simulink model "suduZB"  (R2021a)
settings: Solver=FixedStepAuto  StartTime=0.0  StopTime=20.0  FixedStep=0.01  RelTol=1e-3
libraries: simulink x10
settings Model: Creator=Wang Xu  LastModifiedBy=Wang Xu

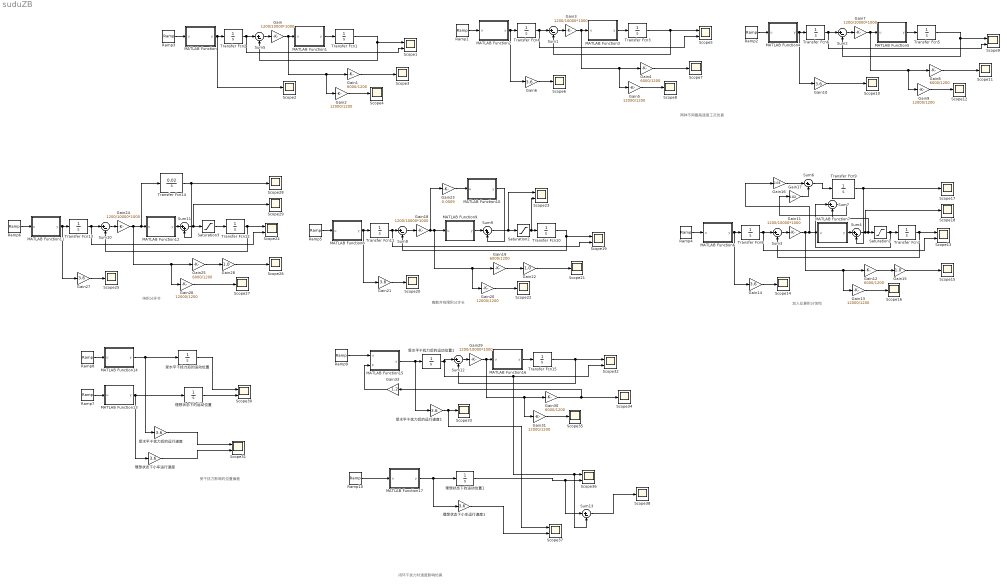
== system suduZB ==
  note: 加入反算积分饱和
  note: 离散并有限积分步长
  note: 纯积分环节
  note: 两种不同最高速度工况仿真
  note: 受干扰力影响的位置偏差
  note: 闭环干扰力对速度影响仿真
  Gain{,3,7,11,18,24,29} (7 alike) : Gain  Gain=1200/10000*1000
  Gain{1,4,8,12,19,25,30} (7 alike) : Gain  Gain=6000/1200
  Gain{6,10,14,21,27} (5 alike) : Gain  Gain=3.6
  Gain{2,5,9,13,20,26,31} (7 alike) : Gain  Gain=12000/1200
  Gain15 : Gain  Gain=1.0
  Gain16 : Gain  Gain=0.03
  Gain17 : Gain  Gain=0.02
  Gain22 : Gain  Gain=1.0
  Gain23 : Gain  Gain=0.0009
  Gain28 : Gain  Gain=1.0
  Gain33 : Gain  Gain=1.2
  MATLAB Function : MATLAB Function  TreatAsAtomicUnit=on
  MATLAB Function1 : MATLAB Function  TreatAsAtomicUnit=on
  MATLAB Function10 : MATLAB Function  TreatAsAtomicUnit=on
  MATLAB Function11 : MATLAB Function  TreatAsAtomicUnit=on
  MATLAB Function12 : MATLAB Function  TreatAsAtomicUnit=on
  MATLAB Function13 : MATLAB Function  TreatAsAtomicUnit=on
  MATLAB Function14 : MATLAB Function  TreatAsAtomicUnit=on
  MATLAB Function15 : MATLAB Function  TreatAsAtomicUnit=on
  MATLAB Function16 : MATLAB Function  TreatAsAtomicUnit=on
  MATLAB Function17 : MATLAB Function  TreatAsAtomicUnit=on
  MATLAB Function2 : MATLAB Function  TreatAsAtomicUnit=on
  MATLAB Function3 : MATLAB Function  TreatAsAtomicUnit=on
  MATLAB Function4 : MATLAB Function  TreatAsAtomicUnit=on
  MATLAB Function5 : MATLAB Function  TreatAsAtomicUnit=on
  MATLAB Function6 : MATLAB Function  TreatAsAtomicUnit=on
  MATLAB Function7 : MATLAB Function  TreatAsAtomicUnit=on
  MATLAB Function8 : MATLAB Function  TreatAsAtomicUnit=on
  MATLAB Function9 : MATLAB Function  TreatAsAtomicUnit=on
  Ramp{1..10} (10 alike) : simulink/Sources/Ramp  slope=1  start=0  InitialOutput=0
  Saturation1 : Saturate  UpperLimit=2.80  LowerLimit=-2.80
  Saturation2 : Saturate  UpperLimit=2.85  LowerLimit=-2.85
  Saturation3 : Saturate  UpperLimit=2.85  LowerLimit=-2.85
  Scope{1,5,9,13,19,23..24,30..32,36..37} (12 alike) : Scope  NumInputPorts=2
  Scope{2..4,6..8,10..12,14..18,20..22,25..29,33..35,38} (26 alike) : Scope
  Sum{1..3,5..8,10,12..13} (10 alike) : Sum  Inputs=|+-
  Sum11 : Sum  Inputs=|++
  Sum4 : Sum  Inputs=|++
  Sum9 : Sum  Inputs=|++
  Transfer Fcn{1..13,15} (14 alike) : TransferFcn  Denominator=[1 0]
  Transfer Fcn14 : TransferFcn  Numerator=[0.02]  Denominator=[1 0]
  受水平干扰力后的运动位置 : TransferFcn  Denominator=[1 0]
  受水平干扰力后的运动位置1 : TransferFcn  Denominator=[1 0]
  受水平干扰力后的运行速度 : Gain  Gain=3.6
  受水平干扰力后的运行速度1 : Gain  Gain=3.6
  理想状态下小车运行速度 : Gain  Gain=3.6
  理想状态下小车运行速度1 : Gain  Gain=3.6
  理想状态下的运动位置 : TransferFcn  Denominator=[1 0]
  理想状态下的运动位置1 : TransferFcn  Denominator=[1 0]
  wires:
  Ramp3/1 -> MATLAB Function/1(u)
  MATLAB Function/1(y) -> Scope2/1, Transfer Fcn2/1
  Transfer Fcn1/1 -> Scope1/1, Sum5/2
  Sum5/1 -> Gain/1
  Transfer Fcn2/1 -> Scope1/2, Sum5/1
  MATLAB Function1/1(y) -> Transfer Fcn1/1
  Gain/1 -> Gain2/1, Gain1/1, MATLAB Function1/1(u)
  Gain1/1 -> Scope3/1
  Gain2/1 -> Scope4/1
  Gain5/1 -> Scope8/1
  Gain4/1 -> Scope7/1
  Transfer Fcn3/1 -> Sum1/2, Scope5/1
  Sum1/1 -> Gain3/1
  Ramp1/1 -> MATLAB Function2/1(u)
  Gain3/1 -> Gain5/1, Gain4/1, MATLAB Function3/1(u)
  Transfer Fcn4/1 -> Scope5/2, Sum1/1
  MATLAB Function3/1(y) -> Transfer Fcn3/1
  MATLAB Function2/1(y) -> Gain6/1, Transfer Fcn4/1
  Gain6/1 -> Scope6/1
  Gain10/1 -> Scope10/1
  Gain8/1 -> Scope11/1
  MATLAB Function4/1(y) -> Gain10/1, Transfer Fcn6/1
  MATLAB Function5/1(y) -> Transfer Fcn5/1
  Transfer Fcn6/1 -> Scope9/2, Sum2/1
  Transfer Fcn5/1 -> Scope9/1, Sum2/2
  Sum2/1 -> Gain7/1
  Gain7/1 -> Gain9/1, Gain8/1, MATLAB Function5/1(u)
  Ramp2/1 -> MATLAB Function4/1(u)
  Gain9/1 -> Scope12/1
  Gain14/1 -> Scope14/1
  Ramp4/1 -> MATLAB Function6/1(u)
  MATLAB Function6/1(y) -> Gain14/1, Transfer Fcn8/1
  Transfer Fcn8/1 -> Scope13/2, Sum3/1
  Gain11/1 -> Gain13/1, Gain12/1, Gain16/1, MATLAB Function7/1(u)
  Gain13/1 -> Scope16/1
  Gain12/1 -> Gain15/1
  Sum3/1 -> Gain11/1
  MATLAB Function7/1(y) -> Sum4/1
  Gain15/1 -> Scope15/1
  Transfer Fcn7/1 -> Sum3/2, Scope13/1
  Sum4/1 -> Scope18/1, Sum7/2, Saturation1/1
  Saturation1/1 -> Sum7/1, Transfer Fcn7/1
  Transfer Fcn9/1 -> Scope17/1, Sum4/2
  Sum6/1 -> Transfer Fcn9/1
  Gain16/1 -> Sum6/1
  Sum7/1 -> Gain17/1
  Gain17/1 -> Sum6/2
  MATLAB Function10/1(y) -> Sum9/2
  Gain23/1 -> MATLAB Function10/1(u)
  MATLAB Function9/1(y) -> Sum9/1
  Transfer Fcn10/1 -> Sum8/2, Scope19/1
  Gain22/1 -> Scope21/1
  Transfer Fcn11/1 -> Scope19/2, Sum8/1
  Sum9/1 -> Scope23/1, Saturation2/1
  Gain19/1 -> Gain22/1
  Saturation2/1 -> Scope23/2, Transfer Fcn10/1
  Sum8/1 -> Gain18/1
  Gain20/1 -> Scope22/1
  Ramp5/1 -> MATLAB Function8/1(u)
  Gain21/1 -> Scope20/1
  MATLAB Function8/1(y) -> Gain21/1, Transfer Fcn11/1
  Gain18/1 -> MATLAB Function9/1(u), Gain20/1, Gain19/1, Gain23/1
  Transfer Fcn14/1 -> Scope28/1, Sum11/2
  Gain24/1 -> Gain26/1, Gain25/1, Transfer Fcn14/1, MATLAB Function12/1(u)
  MATLAB Function12/1(y) -> Sum11/1
  Transfer Fcn12/1 -> Sum10/2, Scope24/1
  Gain28/1 -> Scope26/1
  Transfer Fcn13/1 -> Scope24/2, Sum10/1
  Sum11/1 -> Scope29/1, Saturation3/1
  Gain25/1 -> Gain28/1
  Saturation3/1 -> Transfer Fcn12/1
  Sum10/1 -> Gain24/1
  Ramp6/1 -> MATLAB Function11/1(u)
  Gain27/1 -> Scope25/1
  MATLAB Function11/1(y) -> Gain27/1, Transfer Fcn13/1
  Gain26/1 -> Scope27/1
  Ramp7/1 -> MATLAB Function13/1(u)
  理想状态下小车运行速度/1 -> Scope31/2
  理想状态下的运动位置/1 -> Scope30/2
  MATLAB Function13/1(y) -> 理想状态下小车运行速度/1, 理想状态下的运动位置/1
  Ramp8/1 -> MATLAB Function14/1(u)
  MATLAB Function14/1(y) -> 受水平干扰力后的运动位置/1, 受水平干扰力后的运行速度/1
  受水平干扰力后的运动位置/1 -> Scope30/1
  受水平干扰力后的运行速度/1 -> Scope31/1
  受水平干扰力后的运行速度1/1 -> Scope37/1, Scope33/1
  Transfer Fcn15/1 -> Sum12/2, Scope32/1
  Gain31/1 -> Scope35/1
  Gain30/1 -> Gain33/1, Scope34/1
  MATLAB Function15/1(y) -> 受水平干扰力后的运动位置1/1, 受水平干扰力后的运行速度1/1
  MATLAB Function16/1(y) -> Transfer Fcn15/1
  Gain29/1 -> Gain31/1, Gain30/1, MATLAB Function16/1(u)
  Ramp9/1 -> MATLAB Function15/1(u)
  Sum12/1 -> Gain29/1
  MATLAB Function17/1(y) -> 理想状态下小车运行速度1/1, 理想状态下的运动位置1/1
  理想状态下的运动位置1/1 -> Sum13/1, Scope36/2
  理想状态下小车运行速度1/1 -> Scope37/2
  Ramp10/1 -> MATLAB Function17/1(u)
  受水平干扰力后的运动位置1/1 -> Scope32/2, Sum13/2, Scope36/1, Sum12/1
  Gain33/1 -> MATLAB Function15/2(F)
  Sum13/1 -> Scope38/1

== matlab function suduZB/MATLAB Function14 ==
  data: u input; y output
function y = fcn(u)
v=0;
if u<4.448
    v=0.625*u;
elseif u<10 && u>4.448
    v=2.78;
elseif u<15.4 && u>9.99
    v=2.78-0.6875*(u-10);
else
    v=0;
end

if v<0.0
    v=0.0
end

y = v;

== matlab function suduZB/MATLAB Function15 ==
  data: u input; y output; F input
function y = fcn(u,F)
v=0;
if u<3.78
    v=(1-F/800.0)*u;
elseif u<10 && u>3.78
    v=2.78;
elseif u<15.4 && u>9.99
    v=2.78-1.1*(1.0-F/800.0)*(u-10);
else
    v=0;
end

if v<0.0
    v=0.0
end

if v>2.78
    v=2.78
end

y = v;

== matlab function suduZB/MATLAB Function16 ==
  data: u input; y output
function y = fcn(u)

v=0.0;

if u<6
    v=24*u;
elseif u>6 && u<36
    v=2.5*u*u;
else
    v=90*u;
end
y = v/1000;

== matlab function suduZB/MATLAB Function17 ==
  data: u input; y output
function y = fcn(u)
v=0;
if u<2.78
    v=1*u;
elseif u<10 && u>2.78
    v=2.78;
elseif u<13.4 && u>9.99
    v=2.78-1.1*(u-10);
else
    v=0;
end

if v<0.0
    v=0.0
end

y = v;

== matlab function suduZB/MATLAB Function ==
  data: u input; y output
function y = fcn(u)
v=0;
if u<3.33
    v=1*u;
elseif u<15 && u>3.33
    v=3.33;
elseif u<18 && u>15
    v=3.33-1.1*(u-15);
else
    v=0;
end

y = v;

== matlab function suduZB/MATLAB Function2 ==
  data: u input; y output
function y = fcn(u)
v=0;
if u<2.78
    v=1*u;
elseif u<10 && u>2.78
    v=2.78;
elseif u<12.4 && u>10
    v=2.78-1.1*(u-10);
else
    v=0;
end

y = v;

== matlab function suduZB/MATLAB Function3 ==
  data: u input; y output
function y = fcn(u)

v=0.0;

if u<6
    v=24*u;
elseif u>6 && u<36
    v=2.5*u*u;
else
    v=90*u;
end
y = v/1000;

== matlab function suduZB/MATLAB Function4 ==
  data: u input; y output
function y = fcn(u)
v=0;
if u<4.44
    v=1*u;
elseif u<15 && u>4.44
    v=4.44;
elseif u<19 && u>15
    v=4.44-1.1*(u-15);
else
    v=0;
end

y = v;

== matlab function suduZB/MATLAB Function5 ==
  data: u input; y output
function y = fcn(u)

v=0.0;

if u<6
    v=24*u;
elseif u>6 && u<36
    v=2.5*u*u;
else
    v=90*u;
end
y = v/1000;

== matlab function suduZB/MATLAB Function6 ==
  data: u input; y output
function y = fcn(u)
v=0;
if u<2.78
    v=1*u;
elseif u<10 && u>2.78
    v=2.78;
elseif u<12.4 && u>10
    v=2.78-1.1*(u-10);
else
    v=0;
end

y = v;

== matlab function suduZB/MATLAB Function7 ==
  data: u input; y output
function y = fcn(u)

v=0.0;

if u<6
    v=24*u;
elseif u>6 && u<36
    v=2.5*u*u;
else
    v=90*u;
end
y = v/1000;

== matlab function suduZB/MATLAB Function8 ==
  data: u input; y output
function y = fcn(u)
v=0;
if u<2.78
    v=1*u;
elseif u<10 && u>2.78
    v=2.78;
elseif u<12.4 && u>10
    v=2.78-1.1*(u-10);
else
    v=0;
end

y = v;

== matlab function suduZB/MATLAB Function9 ==
  data: u input; y output
function y = fcn(u)

v=0.0;

if u<6
    v=24*u;
elseif u>6 && u<36
    v=2.5*u*u;
else
    v=90*u;
end
y = v/1000;

== matlab function suduZB/MATLAB Function10 ==
  settings: updateMethod=DISCRETE
  data: u input; y output
function y = fcn(u)

persistent data

if isempty(data)
    data=zeros(1,1000);
end

persistent n

if isempty(n)
    n=1;
else
    n=n+1;
end

if n>100
    n=n-100;
end

data(n)=u;

y=sum(data);

== matlab function suduZB/MATLAB Function1 ==
  data: u input; y output
function y = fcn(u)

v=0.0;

if u<6
    v=24*u;
elseif u>6 && u<36
    v=2.5*u*u;
else
    v=90*u;
end
y = v/1000;

== matlab function suduZB/MATLAB Function11 ==
  data: u input; y output
function y = fcn(u)
v=0;
if u<2.78
    v=1*u;
elseif u<10 && u>2.78
    v=2.78;
elseif u<12.4 && u>10
    v=2.78-1.1*(u-10);
else
    v=0;
end

y = v;

== matlab function suduZB/MATLAB Function12 ==
  data: u input; y output
function y = fcn(u)

v=0.0;

if u<6
    v=24*u;
elseif u>6 && u<36
    v=2.5*u*u;
else
    v=90*u;
end
y = v/1000;

== matlab function suduZB/MATLAB Function13 ==
  data: u input; y output
function y = fcn(u)
v=0;
if u<2.78
    v=1*u;
elseif u<10 && u>2.78
    v=2.78;
elseif u<13.4 && u>9.99
    v=2.78-1.1*(u-10);
else
    v=0;
end

if v<0.0
    v=0.0
end

y = v;
